simulink model "quadPID"  (Simulink 8.4)
settings: Solver=ode3  StartTime=0.0  StopTime=10.0  RelTol=1e-3
libraries: simulink x1
settings Model: Creator=Alexey  LastModifiedBy=Dejan
settings DataIOCC: SignalLoggingSaveFormat=Dataset
settings OptimizationCC: InlineParams=on
settings DebuggingCC: FcnCallInpInsideContextMsg=EnableAllAsError
settings GRTTargetCC: CombineOutputUpdateFcns=on  GRTInterface=off

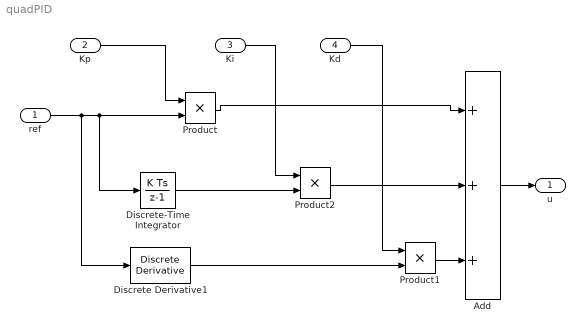
== system quadPID ==
  ref : Inport
  Kp : Inport  Port=2
  Ki : Inport  Port=3
  Kd : Inport  Port=4
  Add : Sum  Inputs=+++
  Discrete Derivative1 : simulink/Discrete/Discrete Derivative  gainval=1.0  ICPrevScaledInput=0.0  InputProcessing=Inherited  OutMin=[]  OutMax=[]  OutDataType=fixdt(1, 16)  OutScaling=2^-10  DoSatur=off
  Discrete-Time Integrator : DiscreteIntegrator  InitialConditionSetting=State (most efficient)  SampleTime=-1
  Product : Product  RndMeth=Zero
  Product1 : Product  RndMeth=Zero
  Product2 : Product  RndMeth=Zero
  u : Outport
  wires:
  Add/1 -> u/1
  Kp/1 -> Product/1
  ref/1 -> Discrete-Time Integrator/1, Product/2, Discrete Derivative1/1
  Product/1 -> Add/1
  Discrete Derivative1/1 -> Product1/2
  Discrete-Time Integrator/1 -> Product2/2
  Product1/1 -> Add/3
  Product2/1 -> Add/2
  Kd/1 -> Product1/1
  Ki/1 -> Product2/1
